simulink library "ctrl_ADRC_angular_rate"  (R2018b)
settings: Solver=VariableStepAuto  StartTime=0.0  StopTime=10.0  RelTol=1e-3
libraries: simulink x2, $bdroot x2
settings Model: Creator=Huitao Lv  LastModifiedBy=Huitao Lv

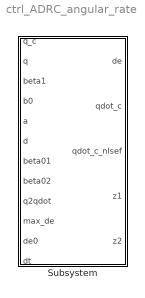
== system ctrl_ADRC_angular_rate ==
  Subsystem : Subsystem  mask(ADRC angular rate controller){}
      mask help: 二阶ADRC姿态角速率控制

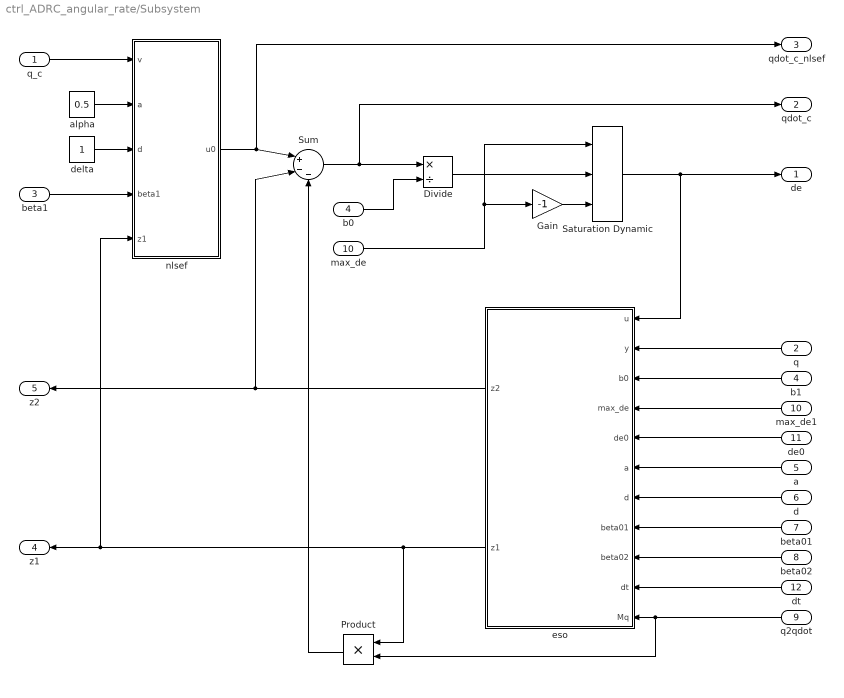
== system ctrl_ADRC_angular_rate/Subsystem ==
  q_c : Inport
  q : Inport  Port=2
  beta1 : Inport  Port=3
  b0 : Inport  Port=4
  a : Inport  Port=5
  d : Inport  Port=6
  beta01 : Inport  Port=7
  beta02 : Inport  Port=8
  q2qdot : Inport  Port=9
  max_de : Inport  Port=10
  de0 : Inport  Port=11
  dt : Inport  Port=12
  Divide : Product  Inputs=*/
  Gain : Gain  Gain=-1
  Product : Product
  Saturation Dynamic : simulink/Discontinuities/Saturation Dynamic  OutMin=[]  OutMax=[]  OutDataTypeStr=Inherit: Same as second input  OutDataType=fixdt(1, 16)  OutScaling=2^-10  DoSatur=off
  Sum : Sum  Inputs=|+--
  alpha : Constant  Value=0.5  OutDataTypeStr=single
  b1 : InportShadow  Port=4
  delta : Constant  OutDataTypeStr=single
  eso : Subsystem  mask(eso){}
      mask help: 二阶带模型信息的扩张状态观测器
  max_de1 : InportShadow  Port=10
  nlsef : Subsystem  mask(nlsef){}
      mask help: 非线性误差反馈控制律
  de : Outport
  qdot_c : Outport  Port=2
  qdot_c_nlsef : Outport  Port=3
  z1 : Outport  Port=4
  z2 : Outport  Port=5
  wires:
  alpha/1 -> nlsef/2(a)
  delta/1 -> nlsef/3(d)
  q_c/1 -> nlsef/1(v)
  beta1/1 -> nlsef/4(beta1)
  nlsef/1(u0) -> qdot_c_nlsef/1, Sum/1
  Sum/1 -> qdot_c/1, Divide/1
  b0/1 -> Divide/2
  Divide/1 -> Saturation Dynamic/2
  max_de/1 -> Saturation Dynamic/1, Gain/1
  Gain/1 -> Saturation Dynamic/3
  Saturation Dynamic/1 -> eso/1(u), de/1
  eso/2(z1) -> Product/1, z1/1, nlsef/5(z1)
  eso/1(z2) -> z2/1, Sum/2
  a/1 -> eso/6(a)
  d/1 -> eso/7(d)
  beta01/1 -> eso/8(beta01)
  beta02/1 -> eso/9(beta02)
  dt/1 -> eso/10(dt)
  q2qdot/1 -> Product/2, eso/11(Mq)
  de0/1 -> eso/5(de0)
  max_de1/1 -> eso/4(max_de)
  b1/1 -> eso/3(b0)
  Product/1 -> Sum/3
  q/1 -> eso/2(y)

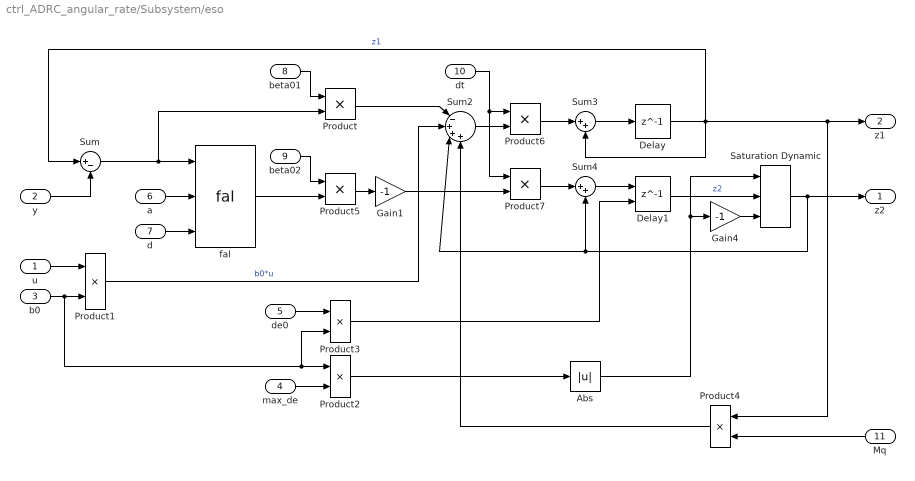
== system ctrl_ADRC_angular_rate/Subsystem/eso ==
  u : Inport
  y : Inport  Port=2
  b0 : Inport  Port=3
  max_de : Inport  Port=4
  de0 : Inport  Port=5
  a : Inport  Port=6
  d : Inport  Port=7
  beta01 : Inport  Port=8
  beta02 : Inport  Port=9
  dt : Inport  Port=10
  Mq : Inport  Port=11
  Abs : Abs
  Delay : Delay  DelayLength=1
  Delay1 : Delay  DelayLength=1  InitialConditionSource=Input port
      settings: InputPortMap=u0,p4
  Gain1 : Gain  Gain=-1
      settings: AttributesFormatString=%<Gain>
  Gain4 : Gain  Gain=-1
  Product{,1..7} (8 alike) : Product
  Saturation Dynamic : simulink/Discontinuities/Saturation Dynamic  OutMin=[]  OutMax=[]  OutDataTypeStr=Inherit: Same as second input  OutDataType=fixdt(1, 16)  OutScaling=2^-10  DoSatur=off
  Sum : Sum  Inputs=|+-
  Sum2 : Sum  Inputs=|-+++
  Sum3 : Sum  Inputs=|++
  Sum4 : Sum  Inputs=|++
  fal : $bdroot/Subsystem/nlsef/fal
  z2 : Outport
  z1 : Outport  Port=2
  wires:
  Abs/1 -> Saturation Dynamic/1, Gain4/1
  de0/1 -> Product3/1
  Sum2/1 -> Product6/2
  Sum3/1 -> Delay/1
  Product/1 -> Sum2/1
  Product2/1 -> Abs/1
  Product3/1 -> Delay1/2
  Saturation Dynamic/1 -> z2/1, Sum2/3, Sum4/2
  Product6/1 -> Sum3/1
  y/1 -> Sum/2
  Product4/1 -> Sum2/4
  b0/1 -> Product1/2, Product2/1, Product3/2
  Gain1/1 -> Product7/2
  Mq/1 -> Product4/2
  Delay/1 -> Sum3/2, Product4/1, z1/1, Sum/1  "z1"
  u/1 -> Product1/1
  max_de/1 -> Product2/2
  d/1 -> fal/3
  Sum/1 -> Product/2, fal/1
  a/1 -> fal/2
  Delay1/1 -> Saturation Dynamic/2  "z2"
  Product1/1 -> Sum2/2  "b0*u"
  Sum4/1 -> Delay1/1
  Product7/1 -> Sum4/1
  beta01/1 -> Product/1
  beta02/1 -> Product5/1
  fal/1 -> Product5/2
  Product5/1 -> Gain1/1
  dt/1 -> Product6/1, Product7/1
  Gain4/1 -> Saturation Dynamic/3

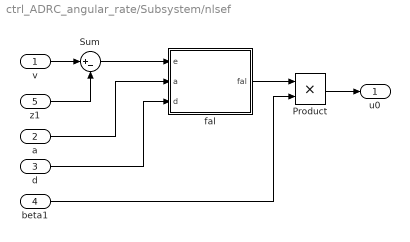
== system ctrl_ADRC_angular_rate/Subsystem/nlsef ==
  v : Inport
  a : Inport  Port=2
  d : Inport  Port=3
  beta1 : Inport  Port=4
  z1 : Inport  Port=5
  Product : Product
  Sum : Sum  Inputs=|+-
  fal : Subsystem  mask(fal){}
      mask help: 最速综合控制函数
  u0 : Outport
  wires:
  z1/1 -> Sum/2
  v/1 -> Sum/1
  Sum/1 -> fal/1(e)
  a/1 -> fal/2(a)
  d/1 -> fal/3(d)
  fal/1(fal) -> Product/1
  beta1/1 -> Product/2
  Product/1 -> u0/1

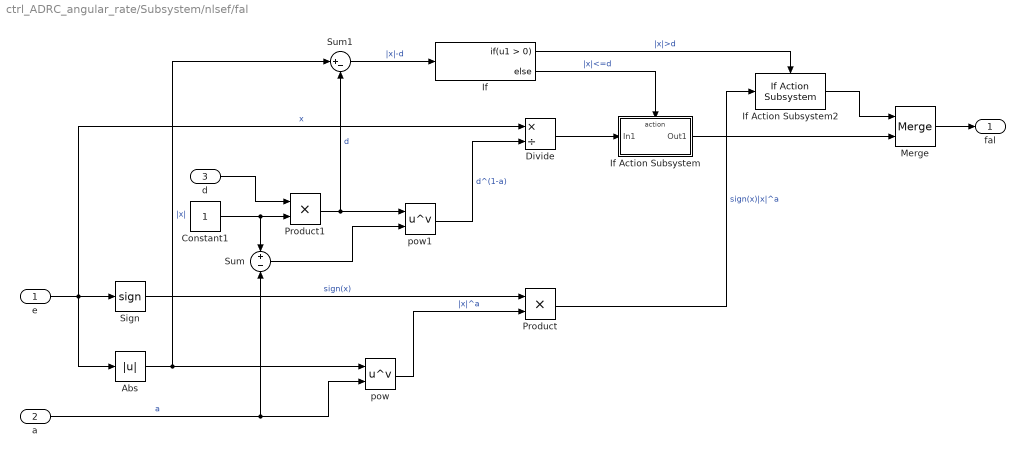
== system ctrl_ADRC_angular_rate/Subsystem/nlsef/fal ==
  e : Inport
  a : Inport  Port=2
  d : Inport  Port=3
  Abs : Abs
  Constant1 : Constant  OutDataTypeStr=single
  Divide : Product  Inputs=*/
  If : If
  If Action Subsystem : Subsystem  TreatAsAtomicUnit=on
  If Action Subsystem2 : $bdroot/Subsystem/nlsef/fal/If Action Subsystem  SystemSampleTime=-1
  Merge : Merge
  Product : Product
  Product1 : Product
  Sign : Signum
  Sum : Sum  Inputs=+-
  Sum1 : Sum  Inputs=|+-
  pow : Math  Operator=pow  SaturateOnIntegerOverflow=on
  pow1 : Math  Operator=pow  SaturateOnIntegerOverflow=on
  fal : Outport
  wires:
  Sign/1 -> Product/1  "sign(x)"
  Divide/1 -> If Action Subsystem/1(In1)
  If Action Subsystem2/1 -> Merge/1
  pow/1 -> Product/2  "|x|^a"
  If/2 -> If Action Subsystem/Action  "|x|<=d"
  Constant1/1 -> Product1/2, Sum/1
  pow1/1 -> Divide/2  "d^(1-a)"
  If/1 -> If Action Subsystem2/Action  "|x|>d"
  Product1/1 -> pow1/1, Sum1/2  "d"
  Sum/1 -> pow1/2
  Merge/1 -> fal/1
  Product/1 -> If Action Subsystem2/1  "sign(x)|x|^a"
  a/1 -> Sum/2, pow/2  "a"
  Sum1/1 -> If/1  "|x|-d"
  If Action Subsystem/1(Out1) -> Merge/2
  Abs/1 -> pow/1, Sum1/1  "|x|"
  e/1 -> Sign/1, Divide/1, Abs/1  "x"
  d/1 -> Product1/1

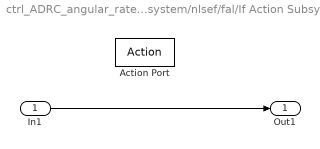
== system ctrl_ADRC_angular_rate/Subsystem/nlsef/fal/If Action Subsystem ==
  In1 : Inport
  Action Port : ActionPort
  Out1 : Outport
  wires:
  In1/1 -> Out1/1
